simulink model "Linearized_observer"  (R2021b)
settings: Solver=VariableStepAuto  StartTime=0.0  StopTime=5  RelTol=1e-3
values from neighbouring files (symbols this model uses):
  eq = [0, 0, pi, 0]    [Linearization_comparison.m]    (also in Synthesis.m = [0, 0, -perturbation, 0]; init.m)
  K = acker(A, B, P)    [Synthesis.m]
  L_obs = temp'    [Synthesis.m]
undefined symbols (not defined in the file or in its folder): A, B, C
settings Model: Creator=brizio  LastModifiedBy=brizio

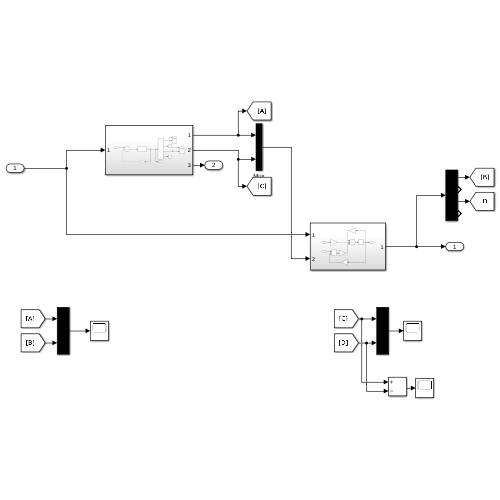
[thumbnail: Simulink's stored preview of the top-level diagram]
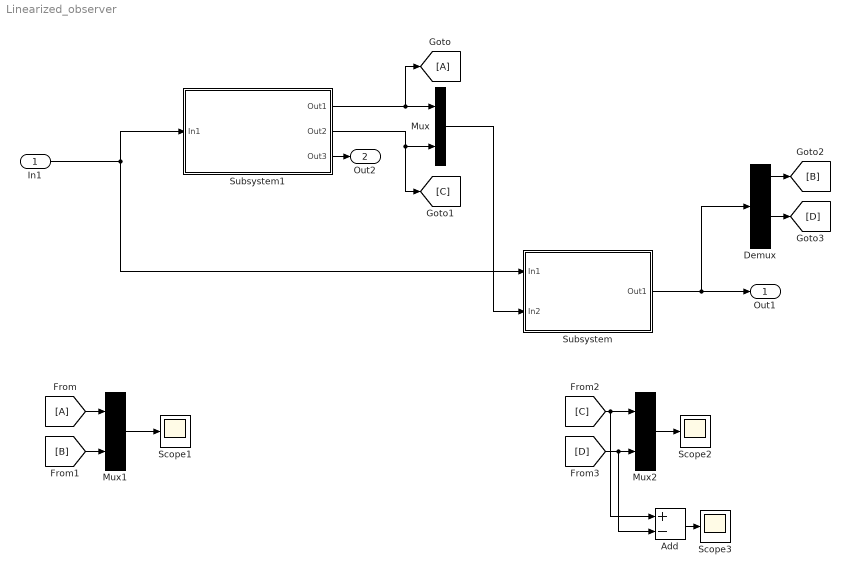
== system Linearized_observer ==
  In1 : Inport
  Add : Sum  Inputs=+-
  Demux : Demux
  Mux : Mux  Inputs=2
  Mux1 : Mux  Inputs=2
  Mux2 : Mux  Inputs=2
  Scope1 : Scope
  Scope2 : Scope
  Scope3 : Scope
  Subsystem : Subsystem
  Subsystem1 : Subsystem
  Out1 : Outport
  Out2 : Outport  Port=2
  wires:
  In1/1 -> Subsystem1/1(In1), Subsystem/1(In1)
  Subsystem/1(Out1) -> Out1/1, Demux/1
  Subsystem1/1(Out1) -> Mux/1, [A]
  Mux/1 -> Subsystem/2(In2)
  Subsystem1/2(Out2) -> [C], Mux/2
  [D] -> Add/2, Mux2/2
  [C] -> Add/1, Mux2/1
  Mux2/1 -> Scope2/1
  Mux1/1 -> Scope1/1
  [A] -> Mux1/1
  [B] -> Mux1/2
  Demux/1 -> [B]
  Demux/3 -> [D]
  Subsystem1/3(Out3) -> Out2/1
  Add/1 -> Scope3/1

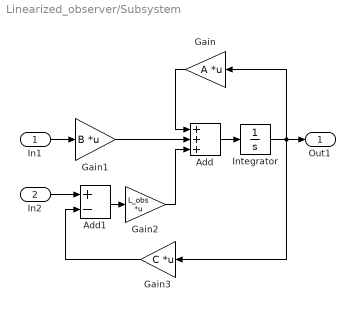
== system Linearized_observer/Subsystem ==
  In1 : Inport
  In2 : Inport  Port=2
  Add : Sum  Inputs=+++
  Add1 : Sum  Inputs=+-
  Gain : Gain  Gain=A  Multiplication=Matrix(K*u)
  Gain1 : Gain  Gain=B  Multiplication=Matrix(K*u)
  Gain2 : Gain  Gain=L_obs  Multiplication=Matrix(K*u)
  Gain3 : Gain  Gain=C  Multiplication=Matrix(K*u)
  Integrator : Integrator
  Out1 : Outport
  wires:
  Add/1 -> Integrator/1
  In1/1 -> Gain1/1
  Gain/1 -> Add/1
  Gain1/1 -> Add/2
  Gain2/1 -> Add/3
  Add1/1 -> Gain2/1
  In2/1 -> Add1/1
  Gain3/1 -> Add1/2
  Integrator/1 -> Gain3/1, Gain/1, Out1/1

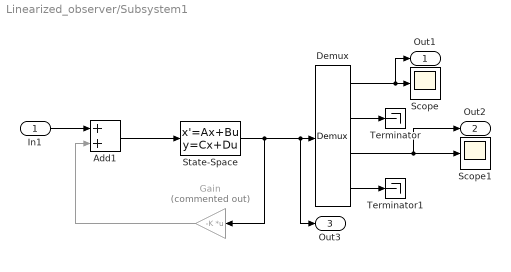
== system Linearized_observer/Subsystem1 ==
  In1 : Inport
  Add1 : Sum
  Demux : Demux
      settings: DisplayOption=none
  Gain : Gain  Commented=on  Gain=-K  Multiplication=Matrix(K*u)
  Scope : Scope
  Scope1 : Scope
  State-Space : StateSpace  A=A  B=B  C=eye(4)  D=zeros(4, 1)  InitialCondition=eq
  Terminator : Terminator
  Terminator1 : Terminator
  Out1 : Outport
  Out2 : Outport  Port=2
  Out3 : Outport  Port=3
  wires:
  Demux/1 -> Out1/1, Scope/1
  Demux/4 -> Terminator1/1
  Demux/3 -> Out2/1, Scope1/1
  State-Space/1 -> Gain/1, Out3/1, Demux/1
  In1/1 -> Add1/1
  Gain/1 -> Add1/2
  Add1/1 -> State-Space/1
  Demux/2 -> Terminator/1
